simulink model "Disturance_behaviour_sim"  (R2018b)
settings: Solver=VariableStepAuto  StartTime=0.0  StopTime=10.0  RelTol=1e-3
PreLoadFcn:
  | % NOTE: If using VoltPAQ-X1, make sure both Gain switches are set to 3.
  | K_AMP = 3;
  | % Maximum Output Voltage (V): YAW limited to 15 V. PITCH limited to 24 V.
  | VMAX_AMP_P = 24;
  | VMAX_AMP_Y = 15;
  | % Initial Angle of Pitch (rad)
  | theta_0 = -40.5*pi/180;
  | 
  | g = 9.81;
  | 
  | % Pitch and Yaw Motor Armature Resistance (Ohm)
  | R_m_p = 0.83;
  | R_m_y = 1.60;
  | 
  | % Pitch and Yaw Motor Current-Torque Constant (N.m/A)
  | K_t_p = 0.0182;
  | K_t_y = 0.0109;
  | 
  | % Pitch and Yaw Motor Voltage-Torque Constant (N.m/V)
  | K_yp = K_t_p / R_m_p;
  | K_py = K_t_y / R_m_y;
  | 
  | % Pitch and Yaw Viscous Damping Constant (N.m.s/rad)
  | B_p = 0.8;  % tuned while running simulation and experiment in parallel
  | B_y = 0.318; % identified as described in manual
  | 
  | % Mass of the Helicopter (kg)
  | m_heli = 1.3872;
  | 
  | % Mass of the Helicopter with Yoke (kg)
  | m_heli_case = 1.421;
  | 
  | % Distance from Pitch Pivot to Pitch/Front Motor and Yaw/Back Motor(m)
  | r_p = 7.75*0.0254;
  | r_y = (6+5/8)*0.0254;
  | 
  | % Pitch and Yaw Propeller Force-Thrust Constant found Experimentally (N/V)
  | K_f_p = 5*0.2074;
  | K_f_y = 3*0.1426;
  | 
  | % Pitch and Yaw Propeller Torque-Thrust Constant found Experimentally (N.m/V)
  | K_pp = K_f_p * r_p;
  | K_yy = K_f_y * r_y;
  | 
  | % Mass of Pitch/Front Motor and Yaw/Back Motor (kg)
  | m_motor_p = 0.292;
  | m_motor_y = 0.128;
  | 
  | % Mass of Pitch/Front and Yaw/Back Guard + Propeller(kg)
  | m_shield = 0.143 + 0.024;
  | 
  | % Total Mass of Pitch and Yaw Motor/Shield Assemblies (kg)
  | m_props = ( m_motor_p + m_motor_y + 2 * m_shield );
  | 
  | % Mass of Helicopter Body moving about Pitch Axis (kg)
  | m_body_p = m_heli - m_props;
  | 
  | % Mass of Helicopter Body moving about Yaw Axis (kg)
  | m_body_y = m_heli_case - m_props;
  | 
  | % Mass of Metal Shaft Moving about Yaw Axis (kg)
  | m_shaft = 0.151;
  | 
  | % Total Length of Helicopter Body (m)
  | L_body = 19*0.0254;
  | 
  | % Helicopter Center of Mass from Pivot along Pitch Axis (m)
  | l_cm = ( (m_motor_p + m_shield ) * r_p +  (m_motor_y + m_shield ) * r_y ) / ( m_props ) ;
  | 
  | % Length of Metal Shaft Moving about Yaw Axis through slip ring (m)
  | L_shaft = 11 * 0.0254;
  | 
  | % Pitch and Yaw Motor Rotor Moment of Inertia (kg.m^2)
  | J_m_p = 1.91e-6; %1.7070e-5;
  | J_m_y = 1.374e-4; %1.4471e-5;
  | 
  | % Moment of Inertia of Helicopter Body about its CM (kg.m^2)
  | J_body_p = m_body_p * L_body^2 / 12;
  | J_body_y = m_body_y * L_body^2 / 12;
  | 
  | % Moment of Inertia of Metal Shaft about Yaw Axis (kg.m^2)
  | J_shaft = m_shaft * L_shaft^2 / 3; %;0.0851;
  | 
  | % Moment of Inertia of Pitch Motor + Guard Assembly about Pivot (kg.m^2)
  | J_p = ( m_motor_p + m_shield ) * r_p^2;
  | 
  | % Moment of Inertia of Yaw Motor + Guard Assembly about Pivot (kg.m^2)
  | J_y = ( m_motor_y + m_shield ) * r_y^2;
  | 
  | % Equivalent Moment of Inertia about Pitch and Yaw Axis (kg.m^2)
  | J_eq_p = J_m_p + J_body_p + J_p + J_y;
  | J_eq_y = J_m_y + J_body_y + J_p + J_y + J_shaft;
  | 
  | 
  | %BESSEL wn=4
  | Kbes=[     68.5119  -25.1203    5.3421   -3.6881
  |    63.1652  188.4894    0.7783   19.4789];
  | 
  | xd=-20;
InitFcn:
  | % NOTE: If using VoltPAQ-X1, make sure both Gain switches are set to 3.
  | K_AMP = 3;
  | % Maximum Output Voltage (V): YAW limited to 15 V. PITCH limited to 24 V.
  | VMAX_AMP_P = 24;
  | VMAX_AMP_Y = 15;
  | % Initial Angle of Pitch (rad)
  | theta_0 = -40.5*pi/180;
  | 
  | g = 9.81;
  | 
  | % Pitch and Yaw Motor Armature Resistance (Ohm)
  | R_m_p = 0.83;
  | R_m_y = 1.60;
  | 
  | % Pitch and Yaw Motor Current-Torque Constant (N.m/A)
  | K_t_p = 0.0182;
  | K_t_y = 0.0109;
  | 
  | % Pitch and Yaw Motor Voltage-Torque Constant (N.m/V)
  | K_yp = K_t_p / R_m_p;
  | K_py = K_t_y / R_m_y;
  | 
  | % Pitch and Yaw Viscous Damping Constant (N.m.s/rad)
  | B_p = 0.8;  % tuned while running simulation and experiment in parallel
  | B_y = 0.318; % identified as described in manual
  | 
  | % Mass of the Helicopter (kg)
  | m_heli = 1.3872;
  | 
  | % Mass of the Helicopter with Yoke (kg)
  | m_heli_case = 1.421;
  | 
  | % Distance from Pitch Pivot to Pitch/Front Motor and Yaw/Back Motor(m)
  | r_p = 7.75*0.0254;
  | r_y = (6+5/8)*0.0254;
  | 
  | % Pitch and Yaw Propeller Force-Thrust Constant found Experimentally (N/V)
  | K_f_p = 5*0.2074;
  | K_f_y = 3*0.1426;
  | 
  | % Pitch and Yaw Propeller Torque-Thrust Constant found Experimentally (N.m/V)
  | K_pp = K_f_p * r_p;
  | K_yy = K_f_y * r_y;
  | 
  | % Mass of Pitch/Front Motor and Yaw/Back Motor (kg)
  | m_motor_p = 0.292;
  | m_motor_y = 0.128;
  | 
  | % Mass of Pitch/Front and Yaw/Back Guard + Propeller(kg)
  | m_shield = 0.143 + 0.024;
  | 
  | % Total Mass of Pitch and Yaw Motor/Shield Assemblies (kg)
  | m_props = ( m_motor_p + m_motor_y + 2 * m_shield );
  | 
  | % Mass of Helicopter Body moving about Pitch Axis (kg)
  | m_body_p = m_heli - m_props;
  | 
  | % Mass of Helicopter Body moving about Yaw Axis (kg)
  | m_body_y = m_heli_case - m_props;
  | 
  | % Mass of Metal Shaft Moving about Yaw Axis (kg)
  | m_shaft = 0.151;
  | 
  | % Total Length of Helicopter Body (m)
  | L_body = 19*0.0254;
  | 
  | % Helicopter Center of Mass from Pivot along Pitch Axis (m)
  | l_cm = ( (m_motor_p + m_shield ) * r_p +  (m_motor_y + m_shield ) * r_y ) / ( m_props ) ;
  | 
  | % Length of Metal Shaft Moving about Yaw Axis through slip ring (m)
  | L_shaft = 11 * 0.0254;
  | 
  | % Pitch and Yaw Motor Rotor Moment of Inertia (kg.m^2)
  | J_m_p = 1.91e-6; %1.7070e-5;
  | J_m_y = 1.374e-4; %1.4471e-5;
  | 
  | % Moment of Inertia of Helicopter Body about its CM (kg.m^2)
  | J_body_p = m_body_p * L_body^2 / 12;
  | J_body_y = m_body_y * L_body^2 / 12;
  | 
  | % Moment of Inertia of Metal Shaft about Yaw Axis (kg.m^2)
  | J_shaft = m_shaft * L_shaft^2 / 3; %;0.0851;
  | 
  | % Moment of Inertia of Pitch Motor + Guard Assembly about Pivot (kg.m^2)
  | J_p = ( m_motor_p + m_shield ) * r_p^2;
  | 
  | % Moment of Inertia of Yaw Motor + Guard Assembly about Pivot (kg.m^2)
  | J_y = ( m_motor_y + m_shield ) * r_y^2;
  | 
  | % Equivalent Moment of Inertia about Pitch and Yaw Axis (kg.m^2)
  | J_eq_p = J_m_p + J_body_p + J_p + J_y;
  | J_eq_y = J_m_y + J_body_y + J_p + J_y + J_shaft;
  | 
  | 
  | %BESSEL wn=4
  | Kbes=[     68.5119  -25.1203    5.3421   -3.6881
  |    63.1652  188.4894    0.7783   19.4789];
  | 
  | xd=-20;
libraries: simulink x1
settings Model: Creator=rezan  LastModifiedBy=rezan
settings DataIOCC: ReturnWorkspaceOutputs=on
settings DebuggingCC: UnconnectedInputMsg=none  UnconnectedOutputMsg=none  UnconnectedLineMsg=none  SFMachineParentedDataDiag=error

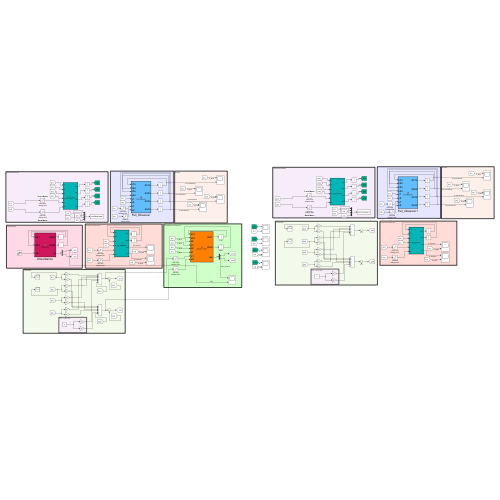
[thumbnail: Simulink's stored preview of the top-level diagram]
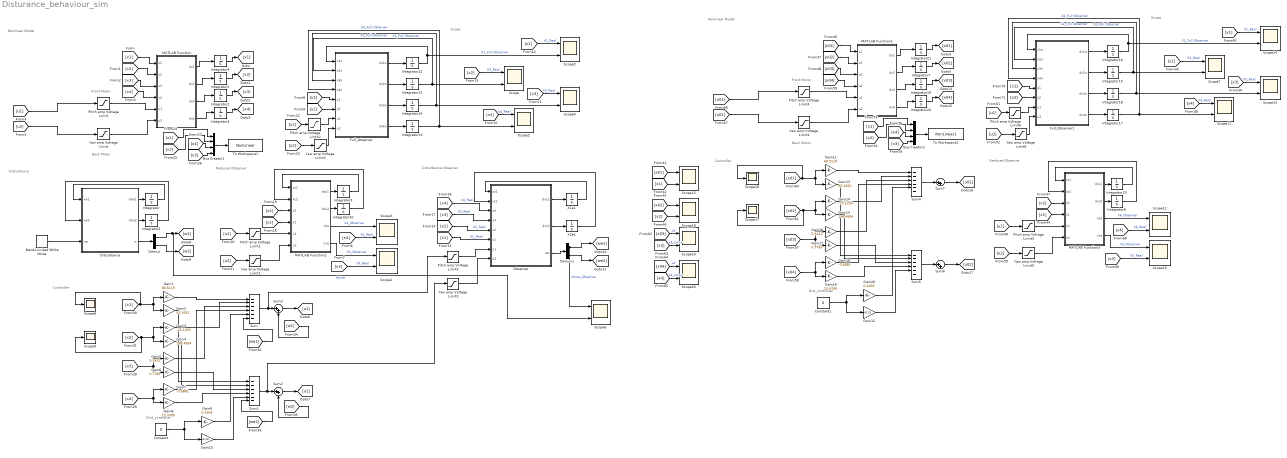
== system Disturance_behaviour_sim ==
  note: Disturbance Observer
  note: Disturbance
  note: Scope
  note: Back Motor
  note: Front Motor
  note: Reduced Observer
  note: Nonlinear Model
  note: Dist_controller
  note: Controller
  note: Scope
  note: Back Motor
  note: Front Motor
  note: Controller
  note: Dist_controller
  note: Reduced Observer
  note: Nonlinear Model
  Band-Limited White Noise : simulink/Sources/Band-Limited White Noise  Cov=[5]  Ts=0.1  seed=[23341]
  Bus Creator1 : BusCreator  Inputs=4
  Bus Creator2 : BusCreator  Inputs=4
  Constant : Constant  Value=0
  Constant1 : Constant  Value=0
  Demux : Demux  Outputs=2
  Demux1 : Demux  Outputs=2
  Disturbance : MATLAB Function  TreatAsAtomicUnit=on
  Full_Observer : MATLAB Function  TreatAsAtomicUnit=on
  Full_Observer1 : MATLAB Function  TreatAsAtomicUnit=on
  Gain1 : Gain  Gain=68.5119
  Gain10 : Gain  Gain=-0.13
  Gain11 : Gain  Gain=68.5119
  Gain12 : Gain  Gain=-0.13
  Gain13 : Gain  Gain=63.1652
  Gain14 : Gain  Gain=-25.1203
  Gain15 : Gain  Gain=188.4894
  Gain16 : Gain  Gain=5.3421
  Gain17 : Gain  Gain=0.7783
  Gain18 : Gain  Gain=-3.6881
  Gain19 : Gain  Gain=19.4789
  Gain2 : Gain  Gain=63.1652
  Gain20 : Gain  Gain=0.4269
  Gain3 : Gain  Gain=-25.1203
  Gain4 : Gain  Gain=188.4894
  Gain5 : Gain  Gain=5.3421
  Gain6 : Gain  Gain=0.7783
  Gain7 : Gain  Gain=-3.6881
  Gain8 : Gain  Gain=19.4789
  Gain9 : Gain  Gain=0.4269
  Integrator{,1,3,5,7..18,20,23} (18 alike) : Integrator
  Integrator19 : Integrator  InitialCondition=5
  Integrator2 : Integrator  InitialCondition=5
  Integrator21 : Integrator  UpperSaturationLimit=40.5*pi/180  LowerSaturationLimit=-40.5*pi/180
  Integrator4 : Integrator  UpperSaturationLimit=40.5*pi/180  LowerSaturationLimit=-40.5*pi/180
  MATLAB Function : MATLAB Function  TreatAsAtomicUnit=on
  MATLAB Function1 : MATLAB Function  TreatAsAtomicUnit=on
  MATLAB Function2 : MATLAB Function  TreatAsAtomicUnit=on
  MATLAB Function3 : MATLAB Function  TreatAsAtomicUnit=on
  Observer : MATLAB Function  TreatAsAtomicUnit=on
  Pitch amp Voltage Limit{,1..6} (7 alike) : Saturate  UpperLimit=VMAX_AMP_P  LowerLimit=- VMAX_AMP_P
  Scope{,1..7,10..15,18..20} (17 alike) : Scope  NumInputPorts=2
  Scope{8..9,16..17} (4 alike) : Scope
  Sum{,1,4..5} (4 alike) : Sum  Inputs=------
  Sum{2..3,6..7} (4 alike) : Sum  Inputs=|++
  To Workspace1 : ToWorkspace  VariableName=NonLinear  SampleTime=-1
  To Workspace2 : ToWorkspace  VariableName=NonLinear1  SampleTime=-1
  X1e1 : Integrator
  X2e1 : Integrator
  Yaw amp Voltage Limit{,1..6} (7 alike) : Saturate  UpperLimit=VMAX_AMP_Y  LowerLimit=- VMAX_AMP_Y
  wires:
  Integrator9/1 -> MATLAB Function2/1(xc1)
  MATLAB Function/2(dx2) -> Integrator1/1
  [u2] -> Yaw amp Voltage Limit/1
  [x2] -> MATLAB Function/2(x2)
  [x4] -> Bus Creator1/3
  Pitch amp Voltage Limit1/1 -> MATLAB Function2/5(u1)
  MATLAB Function2/4(x1e) -> Scope1/1  "X3_Observer"
  Integrator4/1 -> [x1]
  Integrator1/1 -> [x2]
  MATLAB Function/4(dx4) -> Integrator3/1
  [x4] -> MATLAB Function/4(x4)
  Integrator3/1 -> [x4]
  [x1] -> Bus Creator1/1
  [u1] -> Pitch amp Voltage Limit/1
  [x3] -> Scope1/2  "X3_Real"
  [x2] -> Scope/1  "X3_Real"
  Yaw amp Voltage Limit1/1 -> MATLAB Function2/6(u2)
  [u1] -> Pitch amp Voltage Limit1/1
  [x3] -> MATLAB Function/3(x3)
  Integrator2/1 -> [x3]
  MATLAB Function/1(dx1) -> Integrator4/1
  [x3] -> Bus Creator1/4
  Integrator10/1 -> MATLAB Function2/2(xc2)
  [u2] -> Yaw amp Voltage Limit1/1
  Integrator13/1 -> Scope2/2, Full_Observer/4(x4o)  "X4_Full Observer"
  [x1] -> MATLAB Function/1(x1)
  Pitch amp Voltage Limit2/1 -> Full_Observer/7(u1)
  [x2] -> Bus Creator1/2
  [x4] -> Scope3/2  "X4_Real"
  Pitch amp Voltage Limit/1 -> MATLAB Function/5(u1)
  Integrator11/1 -> Scope/2, Full_Observer/2(x2o)  "X2_Full Observer"
  [x1] -> Scope5/1  "X1_Real"
  [x4] -> Scope2/1  "X4_Real"
  MATLAB Function2/1(dxc1) -> Integrator9/1
  Full_Observer/1(dx1o) -> Integrator12/1
  Yaw amp Voltage Limit2/1 -> Full_Observer/8(u2)
  Integrator12/1 -> Scope5/2, Full_Observer/1(x1o)  "X1_Full Observer"
  Yaw amp Voltage Limit/1 -> MATLAB Function/6(u2)
  MATLAB Function2/3(x2e) -> Scope3/1  "X4_Observer"
  Full_Observer/2(dx2o) -> Integrator11/1
  Full_Observer/3(dx3o) -> Integrator14/1
  MATLAB Function/3(dx3) -> Integrator2/1
  Integrator14/1 -> Scope4/2, Full_Observer/3(x3o)  "X3_Full Observer"
  MATLAB Function2/2(dxc2) -> Integrator10/1
  [x1] -> Full_Observer/5(y1)
  [x3] -> Scope4/1  "X3_Real"
  Bus Creator1/1 -> To Workspace1/1
  [x2] -> Full_Observer/6(y2)
  [u1] -> Pitch amp Voltage Limit2/1
  [u2] -> Yaw amp Voltage Limit2/1
  Full_Observer/4(dx4o) -> Integrator13/1
  Observer/1(dxc1) -> X1e1/1
  Disturbance/1(dxw1) -> Integrator/1
  Integrator/1 -> Disturbance/1(xw1)
  Integrator5/1 -> Disturbance/2(xw2)
  Disturbance/2(dxw2) -> Integrator5/1
  X2e1/1 -> Observer/2(xc2)
  X1e1/1 -> Observer/1(xc1)
  Observer/2(dxc2) -> X2e1/1
  Band-Limited White Noise/1 -> Disturbance/3(uw)
  [x1] -> Observer/6(x1)  "X1_Real"
  [x4] -> Observer/3(x4)  "X4_Real"
  [x3] -> Observer/4(x3)  "X3_Real"
  [x2] -> Observer/5(x2)  "X2_Real"
  Gain8/1 -> Sum1/4
  Gain7/1 -> Sum/4
  Gain4/1 -> Sum1/2
  Gain2/1 -> Sum1/1
  Gain10/1 -> Sum1/5
  Gain5/1 -> Sum/3
  Gain6/1 -> Sum1/3
  [x3] -> Gain5/1, Gain6/1
  Gain9/1 -> Sum/5
  [x1] -> Scope8/1, Gain2/1, Gain1/1
  Constant/1 -> Gain10/1, Gain9/1
  [x4] -> Gain8/1, Gain7/1
  [x2] -> Scope9/1, Gain3/1, Gain4/1
  Gain3/1 -> Sum/2
  Gain1/1 -> Sum/1
  Demux/1 -> Scope6/2, [w1]  "Noise"
  Demux/2 -> [w2]
  Demux1/2 -> [we2]
  Demux1/1 -> Scope6/1, [we1]  "Noise_Observer"
  [we1] -> Sum/6
  Sum2/1 -> [u2]
  Sum3/1 -> [u1]
  [w1] -> Sum3/2
  Sum1/1 -> Yaw amp Voltage Limit3/1, Sum2/1
  Sum/1 -> Pitch amp Voltage Limit3/1, Sum3/1
  Pitch amp Voltage Limit3/1 -> Observer/7(u1)
  Yaw amp Voltage Limit3/1 -> Observer/8(u2)
  Disturbance/3(w) -> Demux/1
  Observer/3(we) -> Demux1/1
  [we2] -> Sum1/6
  [x1] -> MATLAB Function2/4(x1)
  [x2] -> MATLAB Function2/3(x2)
  [w2] -> Sum2/2
  Gain19/1 -> Sum5/4
  Gain14/1 -> Sum4/2
  [x02] -> Scope17/1, Gain14/1, Gain15/1
  Sum5/1 -> Sum6/1
  [x01] -> Scope16/1, Gain13/1, Gain11/1
  Gain17/1 -> Sum5/3
  Pitch amp Voltage Limit4/1 -> MATLAB Function1/5(u1)
  Integrator8/1 -> MATLAB Function3/2(xc2)
  Integrator17/1 -> Scope11/2, Full_Observer1/4(x4o)  "X4_Full Observer"
  MATLAB Function3/1(dxc1) -> Integrator23/1
  Sum6/1 -> [u02]
  Sum7/1 -> [u01]
  Gain20/1 -> Sum4/5
  [x2] -> Bus Creator2/2
  [u2] -> Yaw amp Voltage Limit5/1
  Full_Observer1/3(dx3o) -> Integrator18/1
  Gain16/1 -> Sum4/3
  [x3] -> Bus Creator2/4
  Gain11/1 -> Sum4/1
  Gain18/1 -> Sum4/4
  MATLAB Function3/3(x2e) -> Scope12/1  "X4_Observer"
  [x04] -> Gain19/1, Gain18/1
  [x03] -> Gain16/1, Gain17/1
  Yaw amp Voltage Limit4/1 -> MATLAB Function1/6(u2)
  Integrator20/1 -> [x04]
  [x3] -> Scope13/1  "X3_Real"
  Full_Observer1/4(dx4o) -> Integrator17/1
  [x04] -> MATLAB Function1/4(x4)
  Constant1/1 -> Gain12/1, Gain20/1
  [u2] -> Yaw amp Voltage Limit6/1
  MATLAB Function1/3(dx3) -> Integrator19/1
  Integrator16/1 -> Scope14/2, Full_Observer1/1(x1o)  "X1_Full Observer"
  [u1] -> Pitch amp Voltage Limit6/1
  Gain13/1 -> Sum5/1
  Yaw amp Voltage Limit6/1 -> Full_Observer1/8(u2)
  [x2] -> Full_Observer1/6(y2)
  [x4] -> Scope11/1  "X4_Real"
  MATLAB Function3/2(dxc2) -> Integrator8/1
  Bus Creator2/1 -> To Workspace2/1
  [u02] -> Yaw amp Voltage Limit4/1
  [x1] -> Scope14/1  "X1_Real"
  Integrator7/1 -> [x02]
  Full_Observer1/2(dx2o) -> Integrator15/1
  MATLAB Function1/1(dx1) -> Integrator21/1
  [x3] -> Scope10/2  "X3_Real"
  Integrator19/1 -> [x03]
  Integrator15/1 -> Scope7/2, Full_Observer1/2(x2o)  "X2_Full Observer"
  Pitch amp Voltage Limit5/1 -> MATLAB Function3/5(u1)
  [x4] -> Scope12/2  "X4_Real"
  [x02] -> MATLAB Function1/2(x2)
  Pitch amp Voltage Limit6/1 -> Full_Observer1/7(u1)
  [x1] -> Bus Creator2/1
  MATLAB Function1/4(dx4) -> Integrator20/1
  Integrator18/1 -> Scope13/2, Full_Observer1/3(x3o)  "X3_Full Observer"
  Sum4/1 -> Sum7/1
  [x03] -> MATLAB Function1/3(x3)
  [u1] -> Pitch amp Voltage Limit5/1
  MATLAB Function1/2(dx2) -> Integrator7/1
  [u01] -> Pitch amp Voltage Limit4/1
  [x01] -> MATLAB Function1/1(x1)
  [x1] -> Full_Observer1/5(y1)
  Integrator21/1 -> [x01]
  [x2] -> Scope7/1  "X3_Real"
  [x4] -> Bus Creator2/3
  Gain15/1 -> Sum5/2
  [x1] -> MATLAB Function3/4(x1)
  MATLAB Function3/4(x1e) -> Scope10/1  "X3_Observer"
  [x2] -> MATLAB Function3/3(x2)
  Gain12/1 -> Sum5/5
  Yaw amp Voltage Limit5/1 -> MATLAB Function3/6(u2)
  Full_Observer1/1(dx1o) -> Integrator16/1
  Integrator23/1 -> MATLAB Function3/1(xc1)
  [x01] -> Scope15/1
  [x1] -> Scope15/2
  [x2] -> Scope18/2
  [x02] -> Scope18/1
  [x04] -> Scope20/1  "x4"
  [x4] -> Scope20/2  "x4_noisy"
  [x3] -> Scope19/2  "x3_noisy"
  [x03] -> Scope19/1  "x3"

== matlab function Disturance_behaviour_sim/Observer ==
  data: xc1 input; dxc1 output; xc2 input; x4 input; x3 input; x2 input; x1 input; dxc2 output; u1 input; we output; u2 input
function [dxc1,dxc2,we] = Observer_Noise(xc1,xc2,x4,x3,x2,x1,u1,u2)

Ao=[      0         0    1.0000         0
         0         0         0    1.0000
         0         0   -9.2751         0
         0         0         0   -3.4955];
     
Bo=[      0         0
         0         0
    2.3667    0.0790
    0.2410    0.7913];

 
C = [1 0 0 0;0 1 0 0;0 0 1 0;0 0 0 1];
Aw = [0 1;-4 -4];
Cw = [1 0;0 1];
Aee = Aw;
Cs = eye(4);
Ase = Bo*Cw;
Aes = zeros(2,4);
Ass = Ao;
Bs = Bo;
Be = zeros(2,2);
L = [      -0.0000         0   21.2134   -0.8541
    0.0000         0   -8.9879   71.6669];
u=[u1 u2].'
y = [x1;x2;x3;x4];
xs = [x1;x2;x3;x4];
xc = [xc1;xc2];
dxc = (Aee-L*Cs*Ase)*(xc+L*y)+(Aes*inv(Cs)-L*Cs*Ass*inv(Cs))*y+(Be-L*Cs*Bs)*u;
dxc1 = dxc(1);
dxc2 = dxc(2);
Xe = xc+L*y;
we = Cw*Xe+[12;0];

== matlab function Disturance_behaviour_sim/MATLAB Function2 ==
  data: xc1 input; xc2 input; x2 input; x1 input; u1 input; dxc1 output; dxc2 output; x2e output; x1e output; u2 input
function [dxc1,dxc2,x2e,x1e] = Re_Observer(xc1,xc2,x2,x1,u1,u2)

A=[      0         0    1.0000         0
         0         0         0    1.0000
         0         0   -9.2751         0
         0         0         0   -3.4955];
     
B=[      0         0
         0         0
    2.3667    0.0790
    0.2410    0.7913];
C=[  1     0     0     0
     0     1     0     0];

 D=[  0     0
     0     0];

 
C = eye(2,4);
Aee = A(3:4,3:4);
Aes = A(3:4,1:2);
Ase = A(1:2,3:4);
Ass = A(1:2,1:2);

Be = B(3:4,1);
Bs = B(1:2,1);
u=[u1 u2];
Cs = C(1:2,1:2);
L = [   40.7249         0
         0   56.5045];
xc = [xc1;xc2];
y = [x1;x2];
xs = [x1;x2];
dxc = (Aee-L*Cs*Ase)*(xc+L*y)+(Aes*inv(Cs)-L*Cs*Ass*inv(Cs))*y+(Be-L*Cs*Bs)*u;
dxc1 = dxc(1);
dxc2 = dxc(2);
Xe = xc+L*y;
x1e = Xe(1);
x2e = Xe(2);

== matlab function Disturance_behaviour_sim/Full_Observer1 ==
  data: x1o input; dx1o output; x2o input; x3o input; x4o input; dx2o output; dx3o output; dx4o output; y1 input; y2 input; u1 input; u2 input
function [dx1o,dx2o,dx3o,dx4o] = Full_Observer(x1o,x2o,x3o,x4o,y1,y2,u1,u2)

Ao=[      0         0    1.0000         0
         0         0         0    1.0000
         0         0   -9.2751         0
         0         0         0   -3.4955];
     
Bo=[      0         0
         0         0
    2.3667    0.0790
    0.2410    0.7913];
C=[  1     0     0     0
     0     1     0     0];
u=[u1,u2].';
 
p = [-50 -50 -60 -60];
Lo = 1.0e+03 *[  0.1007         0
         0    0.1065
    2.0658         0
         0    2.6277];

xo = [x1o;x2o;x3o;x4o];
yo = C*xo;
y = [y1;y2];
dxo = Ao*xo+Bo*u+Lo*(y-yo);
dx1o = dxo(1);
dx2o = dxo(2);
dx3o = dxo(3);
dx4o = dxo(4);

== matlab function Disturance_behaviour_sim/MATLAB Function1 ==
  data: x1 input; x2 input; x3 input; x4 input; u1 input; dx1 output; u2 input; dx2 output; dx3 output; dx4 output
function [dx1,dx2,dx3,dx4]= NonlinearFunc(x1,x2,x3,x4,u1,u2)
%% Initial Conditions
% Gravitational Constant (m/s^2)
g = 9.81;

% Pitch and Yaw Motor Armature Resistance (Ohm)
R_m_p = 0.83;
R_m_y = 1.60;

% Pitch and Yaw Motor Current-Torque Constant (N.m/A)
K_t_p = 0.0182;
K_t_y = 0.0109;

% Pitch and Yaw Motor Voltage-Torque Constant (N.m/V)
K_yp = K_t_p / R_m_p;
K_py = K_t_y / R_m_y;

% Pitch and Yaw Viscous Damping Constant (N.m.s/rad)
B_p = 0.8;  % tuned while running simulation and experiment in parallel
B_y = 0.318; % identified as described in manual 

% Mass of the Helicopter (kg)
m_heli = 1.3872;

% Mass of the Helicopter with Yoke (kg)
m_heli_case = 1.421;

% Distance from Pitch Pivot to Pitch/Front Motor and Yaw/Back Motor(m)
r_p = 7.75*0.0254;
r_y = (6+5/8)*0.0254;

% Pitch and Yaw Propeller Force-Thrust Constant found Experimentally (N/V)
K_f_p = 5*0.2074;
K_f_y = 3*0.1426;

% Pitch and Yaw Propeller Torque-Thrust Constant found Experimentally (N.m/V)
K_pp = K_f_p * r_p;
K_yy = K_f_y * r_y;

% Mass of Pitch/Front Motor and Yaw/Back Motor (kg)
m_motor_p = 0.292;
m_motor_y = 0.128;

% Mass of Pitch/Front and Yaw/Back Guard + Propeller(kg)
m_shield = 0.143 + 0.024;

% Total Mass of Pitch and Yaw Motor/Shield Assemblies (kg)
m_props = ( m_motor_p + m_motor_y + 2 * m_shield );

% Mass of Helicopter Body moving about Pitch Axis (kg)
m_body_p = m_heli - m_props; 

% Mass of Helicopter Body moving about Yaw Axis (kg)
m_body_y = m_heli_case - m_props; 

% Mass of Metal Shaft Moving about Yaw Axis (kg)
m_shaft = 0.151;

% Total Length of Helicopter Body (m)
L_body = 19*0.0254;

% Helicopter Center of Mass from Pivot along Pitch Axis (m)
l_cm = ( (m_motor_p + m_shield ) * r_p +  (m_motor_y + m_shield ) * r_y ) / ( m_props ) ;

% Length of Metal Shaft Moving about Yaw Axis through slip ring (m)
L_shaft = 11 * 0.0254;

% Pitch and Yaw Motor Rotor Moment of Inertia (kg.m^2)
J_m_p = 1.91e-6; %1.7070e-5;
J_m_y = 1.374e-4; %1.4471e-5;

% Moment of Inertia of Helicopter Body about its CM (kg.m^2)
J_body_p = m_body_p * L_body^2 / 12;
J_body_y = m_body_y * L_body^2 / 12;

% Moment of Inertia of Metal Shaft about Yaw Axis (kg.m^2)
J_shaft = m_shaft * L_shaft^2 / 3; %;0.0851;

% Moment of Inertia of Pitch Motor + Guard Assembly about Pivot (kg.m^2)
J_p = ( m_motor_p + m_shield ) * r_p^2;

% Moment of Inertia of Yaw Motor + Guard Assembly about Pivot (kg.m^2)
J_y = ( m_motor_y + m_shield ) * r_y^2;

% Equivalent Moment of Inertia about Pitch and Yaw Axis (kg.m^2)
J_eq_p = J_m_p + J_body_p + J_p + J_y;
J_eq_y = J_m_y + J_body_y + J_p + J_y + J_shaft;
%%
%%
xd=0
 dx1=x3;
dx2=x4;
dx3=(1/(J_eq_p +m_heli*l_cm^2))*((K_pp*u1+K_py*u2)-(B_p*x3+m_heli*l_cm^2*x4^2*sin(x1)*cos(x1)+m_heli*g*l_cm*cos(x1)));
dx3=dx3+xd;
dx4=1/(J_eq_y + m_heli *l_cm^2* (cos(x1))^2 )*((K_yp*u1 )+(K_yy*u2 ))+(-B_y*x4+2*m_heli*l_cm^2*x4*x3*sin(x1)*cos(x1))/(J_eq_p+ m_heli * l_cm^2 * (cos(x1))^2);

== matlab function Disturance_behaviour_sim/MATLAB Function3 ==
  data: xc1 input; xc2 input; x2 input; x1 input; u1 input; dxc1 output; dxc2 output; x2e output; x1e output; u2 input
function [dxc1,dxc2,x2e,x1e] = Re_Observer(xc1,xc2,x2,x1,u1,u2)

A=[      0         0    1.0000         0
         0         0         0    1.0000
         0         0   -9.2751         0
         0         0         0   -3.4955];
     
B=[      0         0
         0         0
    2.3667    0.0790
    0.2410    0.7913];
C=[  1     0     0     0
     0     1     0     0];

 D=[  0     0
     0     0];

 
C = eye(2,4);
Aee = A(3:4,3:4);
Aes = A(3:4,1:2);
Ase = A(1:2,3:4);
Ass = A(1:2,1:2);

Be = B(3:4,1);
Bs = B(1:2,1);
u=[u1 u2];
Cs = C(1:2,1:2);
L = [   40.7249         0
         0   56.5045];
xc = [xc1;xc2];
y = [x1;x2];
xs = [x1;x2];
dxc = (Aee-L*Cs*Ase)*(xc+L*y)+(Aes*inv(Cs)-L*Cs*Ass*inv(Cs))*y+(Be-L*Cs*Bs)*u;
dxc1 = dxc(1);
dxc2 = dxc(2);
Xe = xc+L*y;
x1e = Xe(1);
x2e = Xe(2);

== matlab function Disturance_behaviour_sim/Full_Observer ==
  data: x1o input; dx1o output; x2o input; x3o input; x4o input; dx2o output; dx3o output; dx4o output; y1 input; y2 input; u1 input; u2 input
function [dx1o,dx2o,dx3o,dx4o] = Full_Observer(x1o,x2o,x3o,x4o,y1,y2,u1,u2)

Ao=[      0         0    1.0000         0
         0         0         0    1.0000
         0         0   -9.2751         0
         0         0         0   -3.4955];
     
Bo=[      0         0
         0         0
    2.3667    0.0790
    0.2410    0.7913];
C=[  1     0     0     0
     0     1     0     0];
u=[u1,u2].';
 
p = [-50 -50 -60 -60];
Lo = 1.0e+03 *[  0.1007         0
         0    0.1065
    2.0658         0
         0    2.6277];

xo = [x1o;x2o;x3o;x4o];
yo = C*xo;
y = [y1;y2];
dxo = Ao*xo+Bo*u+Lo*(y-yo);
dx1o = dxo(1);
dx2o = dxo(2);
dx3o = dxo(3);
dx4o = dxo(4);

== matlab function Disturance_behaviour_sim/MATLAB Function ==
  data: x1 input; x2 input; x3 input; x4 input; u1 input; dx1 output; u2 input; dx2 output; dx3 output; dx4 output
function [dx1,dx2,dx3,dx4]= NonlinearFunc(x1,x2,x3,x4,u1,u2)
%% Initial Conditions
% Gravitational Constant (m/s^2)
g = 9.81;

% Pitch and Yaw Motor Armature Resistance (Ohm)
R_m_p = 0.83;
R_m_y = 1.60;

% Pitch and Yaw Motor Current-Torque Constant (N.m/A)
K_t_p = 0.0182;
K_t_y = 0.0109;

% Pitch and Yaw Motor Voltage-Torque Constant (N.m/V)
K_yp = K_t_p / R_m_p;
K_py = K_t_y / R_m_y;

% Pitch and Yaw Viscous Damping Constant (N.m.s/rad)
B_p = 0.8;  % tuned while running simulation and experiment in parallel
B_y = 0.318; % identified as described in manual 

% Mass of the Helicopter (kg)
m_heli = 1.3872;

% Mass of the Helicopter with Yoke (kg)
m_heli_case = 1.421;

% Distance from Pitch Pivot to Pitch/Front Motor and Yaw/Back Motor(m)
r_p = 7.75*0.0254;
r_y = (6+5/8)*0.0254;

% Pitch and Yaw Propeller Force-Thrust Constant found Experimentally (N/V)
K_f_p = 5*0.2074;
K_f_y = 3*0.1426;

% Pitch and Yaw Propeller Torque-Thrust Constant found Experimentally (N.m/V)
K_pp = K_f_p * r_p;
K_yy = K_f_y * r_y;

% Mass of Pitch/Front Motor and Yaw/Back Motor (kg)
m_motor_p = 0.292;
m_motor_y = 0.128;

% Mass of Pitch/Front and Yaw/Back Guard + Propeller(kg)
m_shield = 0.143 + 0.024;

% Total Mass of Pitch and Yaw Motor/Shield Assemblies (kg)
m_props = ( m_motor_p + m_motor_y + 2 * m_shield );

% Mass of Helicopter Body moving about Pitch Axis (kg)
m_body_p = m_heli - m_props; 

% Mass of Helicopter Body moving about Yaw Axis (kg)
m_body_y = m_heli_case - m_props; 

% Mass of Metal Shaft Moving about Yaw Axis (kg)
m_shaft = 0.151;

% Total Length of Helicopter Body (m)
L_body = 19*0.0254;

% Helicopter Center of Mass from Pivot along Pitch Axis (m)
l_cm = ( (m_motor_p + m_shield ) * r_p +  (m_motor_y + m_shield ) * r_y ) / ( m_props ) ;

% Length of Metal Shaft Moving about Yaw Axis through slip ring (m)
L_shaft = 11 * 0.0254;

% Pitch and Yaw Motor Rotor Moment of Inertia (kg.m^2)
J_m_p = 1.91e-6; %1.7070e-5;
J_m_y = 1.374e-4; %1.4471e-5;

% Moment of Inertia of Helicopter Body about its CM (kg.m^2)
J_body_p = m_body_p * L_body^2 / 12;
J_body_y = m_body_y * L_body^2 / 12;

% Moment of Inertia of Metal Shaft about Yaw Axis (kg.m^2)
J_shaft = m_shaft * L_shaft^2 / 3; %;0.0851;

% Moment of Inertia of Pitch Motor + Guard Assembly about Pivot (kg.m^2)
J_p = ( m_motor_p + m_shield ) * r_p^2;

% Moment of Inertia of Yaw Motor + Guard Assembly about Pivot (kg.m^2)
J_y = ( m_motor_y + m_shield ) * r_y^2;

% Equivalent Moment of Inertia about Pitch and Yaw Axis (kg.m^2)
J_eq_p = J_m_p + J_body_p + J_p + J_y;
J_eq_y = J_m_y + J_body_y + J_p + J_y + J_shaft;
%%
%%
xd=0
 dx1=x3;
dx2=x4;
dx3=(1/(J_eq_p +m_heli*l_cm^2))*((K_pp*u1+K_py*u2)-(B_p*x3+m_heli*l_cm^2*x4^2*sin(x1)*cos(x1)+m_heli*g*l_cm*cos(x1)));
dx3=dx3+xd;
dx4=1/(J_eq_y + m_heli *l_cm^2* (cos(x1))^2 )*((K_yp*u1 )+(K_yy*u2 ))+(-B_y*x4+2*m_heli*l_cm^2*x4*x3*sin(x1)*cos(x1))/(J_eq_p+ m_heli * l_cm^2 * (cos(x1))^2);

== matlab function Disturance_behaviour_sim/Disturbance ==
  data: xw1 input; dxw1 output; xw2 input; dxw2 output; w output; uw input
function [dxw1,dxw2,w] = Disturbance(xw1,xw2,uw)

Aw = [0 1;-4 -4];
xw = [xw1;xw2]+[0;1]*uw;
dxw = Aw*xw;
dxw1 = dxw(1);
dxw2 = dxw(2);
Cw = [1 0;0 1];
w = Cw*xw;
